simulink library "librnew"  (Simulink 4.00)
undefined symbols (not defined in the file or in its folder): eyediasi, eyesampl, sbiterr, seed

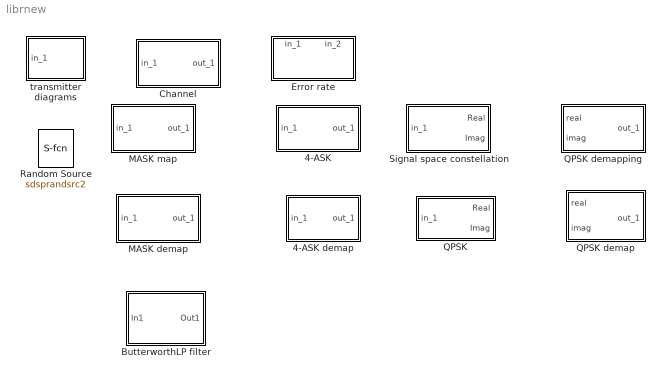
== system librnew ==
  4-ASK : Subsystem  mask(M-ASK mapping){N=4, td=1}
      mask prompts: N "M-ary number (input integers in range [0, M-1]):"; td "Input symbol interval and offset (sec):"
      mask help:
      | Map a digital symbol onto an analog
      | signal in the range [-1, 1] using M-ary
      | amplitude shift keying modulation mapping.
      mask init:
      | Ac=1;Kc=Ac*2/(N-1);
      settings: RTWFcnNameOpts=Auto  RTWFileNameOpts=Auto
      mask Help: This block maps an input digit signal onto a signal in the range [-1, 1]. The coded signal can be modulated using analog\nmodulation blocks. Input digits are in the range [0, M-1], where M is the M-ary number. The input symbol interval can be a two-element vector with the second element being offset. The default value offset is 0. Use the MODMAP function to see the constellation.
      mask Display: disp('MASK\nmapping')
  4-ASK demap : Subsystem  mask(MASK demapping){N=4, td=[1, .9]}
      mask prompts: N "M-ary number (digit integers in ranger [0, M-1]):"; td "Output symbol interval and offset (sec):"
      mask help:
      | Reverse the MASK mapping process
      | Convert [-1 1] analog signal to [0, M-1] symbols.
      mask init:
      | Ac=1;sft=[0:N-1]*Ac*2/(N-1)-Ac;
      settings: RTWFcnNameOpts=Auto  RTWFileNameOpts=Auto
      mask Help: This block demaps a MASK mapped signal back to digit symbols. You can place this block after a amplitude demodulation block. The input of this block is an analog signal in the range [-1, 1]. The demodulation decides the closest integer fitting in [0,M-1] range. When the input symbol interval is a two-elements vector, the second element is offset. The default offset value is 0.
      mask Display: disp('MASK\ndemapping')
  ButterworthLP filter : Subsystem  mask(Lowpass Butterworth filter){n=4}
      mask prompts: n "Cutoff frequency (rad/s)"
      mask init:
      | z = @1 * [];
      | p = @1 * exp(i*(pi*(1:2:n-1)/(2*n) + pi/2));
      | p = [p; conj(p)];
      | p = p(:);
      | if rem(n,2)==1   % n is odd
      |     p = [p; -1];
      | end
      | k = real(prod(-p));
      settings: RTWFcnNameOpts=Auto  RTWFileNameOpts=Auto
      mask Display: plot(0,0,100,100,[90,10,10],[10,10,90],[70,40,9],[10,70,70])
  Channel : Subsystem  mask(AWGN channel, fixed parameter){m=0, variance=0.00010, s=12345}
      mask prompts: m "Mean value:"; variance "Variance (std^2):"; s "Initial Seed:"
      mask help:
      | Additive white Gaussian noise channel
      | with fixed mean and variance.
      mask init:
      | [m,variance,s]=gwnoise(m,variance,s);
      settings: RTWFcnNameOpts=Auto  RTWFileNameOpts=Auto
      mask Help: This block adds white Gaussian noise to the input signal. The mean and the variance can be a scalar or vector with the same length as the input signal.
      mask Display:
      | plot(0,0,100,100);
      | disp('AWGN')
  Error rate : Subsystem  Orientation=down  LoadFcn=sbiterr([],[],[],'LoadBlock')  StartFcn=sbiterr([],[],[],'Start')  StopFcn=sbiterr([],[],[],'Stop')  mask(Symbol/bit error counter){@1=1, @2=10, @3=12, @4=1}
      mask prompts: @1 "Bit per symbol:"; @2 "Number of digits on display:"; @3 "Delay between 1st port and 2nd port:"; @4 "Sample time (sec):"
      mask help: Use the input data from the 1st port as the reference signal to detect the number of errors and error rate of the 2nd signal.
      mask init:
      | K=@1;num_lin=@2;TDelay=@3;Sample=@4;
      settings: CopyFcn=sbiterr([],[],[],'CopyBlock')  DeleteFcn=sbiterr([],[],[],'DeleteBlock')  NameChangeFcn=sbiterr([],[],[],'NameChange')  RTWFcnNameOpts=Auto  RTWFileNameOpts=Auto
      mask Help: The signal from the first port must be a scalar. The second input port can be a vector with a delay to the first port signal. The comparison happens only at the sampling point.
      mask Display: disp('Error\nmeter')
  MASK demap : Subsystem  mask(MASK demap){@1=4, @2=[1, .9]}
      mask prompts: @1 "M-ary number (digit integers in ranger [0, M-1]):"; @2 "Output symbol interval and offset (sec):"
      mask help:
      | Reverse the MASK mapping process
      | Convert [-1 1] analog signal to [0, M-1] symbols.
      mask init:
      | N=@1;Ac=1;sft=[0:N-1]*Ac*2/(N-1)-Ac;td=@2;
      settings: RTWFcnNameOpts=Auto  RTWFileNameOpts=Auto
      mask Help: This block demaps a MASK mapped signal back to digit symbols. You can place this block after a amplitude demodulation block. The input of this block is an analog signal in the range [-1, 1]. The demodulation decides the closest integer fitting in [0,M-1] range. When the input symbol interval is a two-elements vector, the second element is offset. The default offset value is 0.
      mask Display: disp('MASK\ndemap')
  MASK map : Subsystem  mask(MASK map){@1=4, @2=1}
      mask prompts: @1 "M-ary number (input integers in range [0, M-1]):"; @2 "Input symbol interval and offset (sec):"
      mask help:
      | Map a digital symbol onto an analog
      | signal in the range [-1, 1] using M-ary
      | amplitude shift keying modulation mapping.
      mask init:
      | N=@1;Ac=1;Kc=Ac*2/(N-1);td=@2;
      settings: RTWFcnNameOpts=Auto  RTWFileNameOpts=Auto
      mask Help: This block maps an input digit signal onto a signal in the range [-1, 1]. The coded signal can be modulated using analog\nmodulation blocks. Input digits are in the range [0, M-1], where M is the M-ary number. The input symbol interval can be a two-element vector with the second element being offset. The default value offset is 0. Use the MODMAP function to see the constellation.
      mask Display: disp('MASK\nmap')
  QPSK : Subsystem  mask(MPSK){N=[4], A=[sqrt(2)], P=[pi/4], td=1}
      mask prompts: N "Number of symbols in each circle NIC:"; A "Radii in each circle RIC:"; P "Phase shift in each circle PIC (rad):"; td "Symbol interval and offset (sec):"
      mask help: QASK mapping with circle constellation. The constellation is defined in NIC, RIC and PIC.
      mask init:
      | y1=apkconst(N,A,P);y1=[y1;y1];y1=y1(:);y2=imag(y1);y1=real(y1);x=[-sum(N) 1:sum(N)-1;1:sum(N)-1 10*sum(N)]-.5;x=x(:);
      settings: RTWFcnNameOpts=Auto  RTWFileNameOpts=Auto
      mask Help: This block maps a digital signal onto in-phase and quadratic components, which are outputs in the first and second output port respectively. The circle constellation is defined in NIC, RIC, and PIC. The input symbol interval can be a two-element vector with the second element being offset. The default value offset is 0. Use the MODMAP function to see the constellation.
      mask Display: disp('MPSK\nmapping')
  QPSK demap : Subsystem  mask(MPSK demapping){N=[4], A=[sqrt(2)], P=[pi/4], td=1}
      mask prompts: N "Number of symbols on each circle NIC::"; A "Radii for each circle RIC:"; P "Phase shift on each circle PIC (rad):"; td "Symbol interval and offset (sec):"
      mask help:
      | Reverse the QASK map. Input in-phase
      | and quadrature components from the
      | two inputs. Output demapped signal.
      mask init:
      | y1=apkconst(N,A,P);y2=imag(y1);y1=real(y1);
      settings: RTWFcnNameOpts=Auto  RTWFileNameOpts=Auto
      mask Help: This block demaps a QASK mapped signal using circle constellation. You can place this block after a QAM demodulation block. The circle constellation is defined in NIC, RIC, and PIC. The symbol interval can be a two elements vector with the first element being offset. The default offset is zero. Use function MODMAP to view the constellation.
      mask Display: disp('MPSK\ndemapping')
  QPSK demapping : Subsystem  mask(QASK C-demap){@1=[4], @2=[sqrt(2)], @3=[pi/4], @4=1}
      mask prompts: @1 "Number of symbols on each circle NIC::"; @2 "Radii for each circle RIC:"; @3 "Phase shift on each circle PIC (rad):"; @4 "Symbol interval and offset (sec):"
      mask help:
      | Reverse the QASK map. Input in-phase
      | and quadrature components from the
      | two inputs. Output demapped signal.
      mask init:
      | N=@1;A=@2;P=@3;td=@4;y1=apkconst(N,A,P);y2=imag(y1);y1=real(y1);
      settings: RTWFcnNameOpts=Auto  RTWFileNameOpts=Auto
      mask Help: This block demaps a QASK mapped signal using circle constellation. You can place this block after a QAM demodulation block. The circle constellation is defined in NIC, RIC, and PIC. The symbol interval can be a two elements vector with the first element being offset. The default offset is zero. Use function MODMAP to view the constellation.
      mask Display: disp('QASK\nC-demap')
  Random Source : S-Function  FunctionName=sdsprandsrc2  Parameters=SrcType,Min,Max,Mean,Var,SFcnSeed,Inherit,SampMode,SampTime,SampFrame,OutComplex,RepMode,Seed  PortCounts=[]  SFunctionModules=''  mask(Random Source){SrcType=Gaussian, Min=0, Max=1, Mean=0, Var=1, RepMode=Specify seed, Seed=seed, Inherit=on, SampMode=Discrete, SampTime=1, SampFrame=1, OutComplex=Real}
      mask prompts: SrcType "Source type:"; Min "Minimum:"; Max "Maximum:"; Var "Variance:"; RepMode "Repeatability:"; Seed "Initial seed:"; Inherit "Inherit output port attributes"; SampMode "Sample mode:"; SampTime "Sample time:"; SampFrame "Samples per frame:"; OutComplex "Output complexity:"
      mask help: Output a random signal with uniform or Gaussian (normal) distribution. Set output repeatability to Nonrepeatable (block randomly selects initial seed every time simulation starts), Repeatable (block randomly selects initial seed once and uses it every time simulation starts), or Specify seed (block uses specified initial seed every time simulation starts, producing repeatable output).
      mask init:
      | [x,y]=dspblkrandsrc2('icon');SFcnSeed=eval(dspblkrandsrc2('seed'),'Seed');
      mask Help: web(dspbhelp);
      mask StyleString: popup(Uniform|Gaussian),edit,edit,edit,edit,popup(Specify seed|Repeatable|Not repeatable),edit,checkbox,popup(Discrete|Continuous),edit,edit,popup(Real|Complex)
      mask CallbackString: dspblkrandsrc2;|||||dspblkrandsrc2;||dspblkrandsrc2;|dspblkrandsrc2;|||
      mask Display: plot(x,y);
  Signal space constellation : Subsystem  mask(QASK C-map){@1=[4], @2=[sqrt(2)], @3=[pi/4], @4=1}
      mask prompts: @1 "Number of symbols in each circle NIC:"; @2 "Radii in each circle RIC:"; @3 "Phase shift in each circle PIC (rad):"; @4 "Symbol interval and offset (sec):"
      mask help: QASK mapping with circle constellation. The constellation is defined in NIC, RIC and PIC.
      mask init:
      | N=@1;A=@2;P=@3;td=@4;y1=apkconst(N,A,P);y1=[y1;y1];y1=y1(:);y2=imag(y1);y1=real(y1);x=[-sum(N) 1:sum(N)-1;1:sum(N)-1 10*sum(N)]-.5;x=x(:);
      settings: RTWFcnNameOpts=Auto  RTWFileNameOpts=Auto
      mask Help: This block maps a digital signal onto in-phase and quadratic components, which are outputs in the first and second output port respectively. The circle constellation is defined in NIC, RIC, and PIC. The input symbol interval can be a two-element vector with the second element being offset. The default value offset is 0. Use the MODMAP function to see the constellation.
      mask Display: disp('QASK\nC-map')
  transmitter diagrams : Subsystem  mask(Diagrams){starttime=6, anzahl=40, offset=0}
      mask prompts: starttime "Plot start time:"; anzahl "samples per time slot"; offset "decision offset"
      mask help: Eye pattern, signal-space trajectory and scatter plot
      mask init:
      | [x, y] = srcsicon(10);
      settings: RTWFcnNameOpts=Auto  RTWFileNameOpts=Auto
      mask Display: plot(0,0,100,100,x,y)

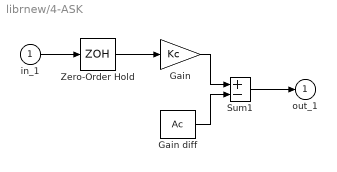
== system librnew/4-ASK ==
  in_1 : Inport  Port=1  LatchInput=off
  Gain : Gain  Gain=Kc  Multiplication=Element-wise(K.*u)  SaturateOnIntegerOverflow=on
  Gain diff : Constant  Value=Ac
  Sum1 : Sum  Inputs=+-  SaturateOnIntegerOverflow=on
  Zero-Order Hold : ZeroOrderHold  SampleTime=td
  out_1 : Outport  Port=1
  wires:
  Gain/1 -> Sum1/1
  Gain diff/1 -> Sum1/2
  Sum1/1 -> out_1/1
  in_1/1 -> Zero-Order Hold/1
  Zero-Order Hold/1 -> Gain/1

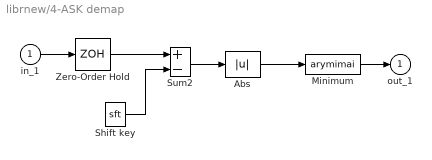
== system librnew/4-ASK demap ==
  in_1 : Inport  Port=1  LatchInput=off
  Abs : Abs  SaturateOnIntegerOverflow=on
  Minimum : S-Function  FunctionName=arymimai  Parameters='min'  PortCounts=[]  SFunctionModules=''
  Shift key : Constant  Value=sft
  Sum2 : Sum  Inputs=+-  SaturateOnIntegerOverflow=on
  Zero-Order Hold : ZeroOrderHold  SampleTime=td
  out_1 : Outport  Port=1
  wires:
  in_1/1 -> Zero-Order Hold/1
  Abs/1 -> Minimum/1
  Zero-Order Hold/1 -> Sum2/1
  Minimum/1 -> out_1/1
  Shift key/1 -> Sum2/2
  Sum2/1 -> Abs/1

== system librnew/ButterworthLP filter ==
  In1 : Inport  Port=1  LatchInput=off
  Zero-Pole : ZeroPole  Zeros=z  Poles=p  Gain=k  AbsoluteTolerance=auto
  Out1 : Outport  Port=1
  wires:
  Zero-Pole/1 -> Out1/1
  In1/1 -> Zero-Pole/1

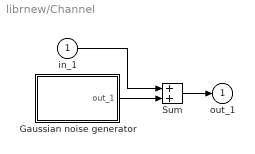
== system librnew/Channel ==
  in_1 : Inport  Port=1  LatchInput=off
  Gaussian noise generator : Subsystem  mask(Gaussian noise generator){m=m, variance=variance, s=s}
      mask prompts: m "Mean value:"; variance "Variance (vector or matrix):"; s "Initial seed:"
      mask help:
      | Generate Gaussian distributed noise with
      | given mean and variance value.
      mask init:
      | [m,variance,s]=gwnoise(m,variance,s);[x,y]=srcsicon(3);
      settings: RTWFcnNameOpts=Auto  RTWFileNameOpts=Auto
      mask Help: When the mean value and seed are vectors, the output of this block is a vector. The length of the vector is the same as the length of the mean value vector or the length of the seed. When the variance entry is a vector, the variance is a diagonal matrix.
      mask Display: plot(0,0,100,100,x,y);disp('Gaussian')
  Sum : Sum  Inputs=++  SaturateOnIntegerOverflow=on
  out_1 : Outport  Port=1
  wires:
  Sum/1 -> out_1/1
  in_1/1 -> Sum/1
  Gaussian noise generator/1(out_1) -> Sum/2

== system librnew/Error rate ==
  in_1 : Inport  Port=1  LatchInput=off
  in_2 : Inport  Port=2  LatchInput=off
  Mux : Mux  Inputs=2
      settings: DisplayOption=none
  S-function : S-Function  FunctionName=sbiterr  Parameters=num_lin, K, TDelay, Sample  PortCounts=[]  SFunctionModules=''
  wires:
  Mux/1 -> S-function/1
  in_1/1 -> Mux/1
  in_2/1 -> Mux/2

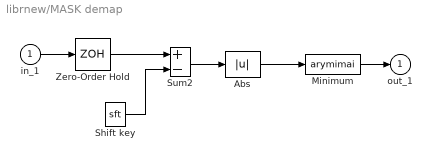
== system librnew/MASK demap ==
  in_1 : Inport  Port=1  LatchInput=off
  Abs : Abs  SaturateOnIntegerOverflow=on
  Minimum : S-Function  FunctionName=arymimai  Parameters='min'  PortCounts=[]  SFunctionModules=''
  Shift key : Constant  Value=sft
  Sum2 : Sum  Inputs=+-  SaturateOnIntegerOverflow=on
  Zero-Order Hold : ZeroOrderHold  SampleTime=td
  out_1 : Outport  Port=1
  wires:
  in_1/1 -> Zero-Order Hold/1
  Abs/1 -> Minimum/1
  Zero-Order Hold/1 -> Sum2/1
  Minimum/1 -> out_1/1
  Shift key/1 -> Sum2/2
  Sum2/1 -> Abs/1

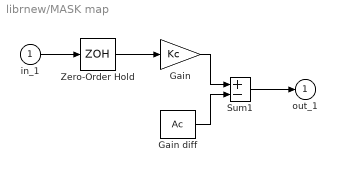
== system librnew/MASK map ==
  in_1 : Inport  Port=1  LatchInput=off
  Gain : Gain  Gain=Kc  Multiplication=Element-wise(K.*u)  SaturateOnIntegerOverflow=on
  Gain diff : Constant  Value=Ac
  Sum1 : Sum  Inputs=+-  SaturateOnIntegerOverflow=on
  Zero-Order Hold : ZeroOrderHold  SampleTime=td
  out_1 : Outport  Port=1
  wires:
  Gain/1 -> Sum1/1
  Gain diff/1 -> Sum1/2
  Sum1/1 -> out_1/1
  in_1/1 -> Zero-Order Hold/1
  Zero-Order Hold/1 -> Gain/1

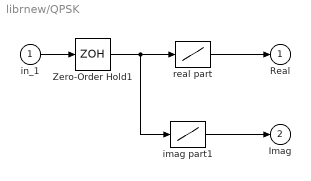
== system librnew/QPSK ==
  in_1 : Inport  Port=1  LatchInput=off
  Zero-Order Hold1 : ZeroOrderHold  SampleTime=td
  imag part1 : Lookup  InputValues=x  OutputValues=y2
  real part : Lookup  InputValues=x  OutputValues=y1
  Real : Outport  Port=1
  Imag : Outport  Port=2
  wires:
  in_1/1 -> Zero-Order Hold1/1
  Zero-Order Hold1/1 -> real part/1, imag part1/1
  real part/1 -> Real/1
  imag part1/1 -> Imag/1

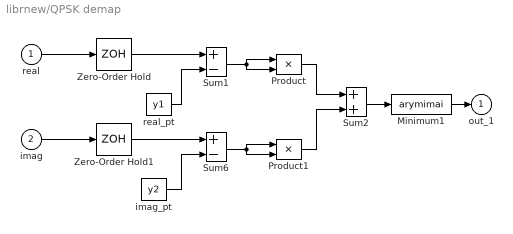
== system librnew/QPSK demap ==
  real : Inport  Port=1  LatchInput=off
  imag : Inport  Port=2  LatchInput=off
  Minimum1 : S-Function  FunctionName=arymimai  Parameters='min'  PortCounts=[]  SFunctionModules=''
  Product : Product  Inputs=2  Multiplication=Element-wise(.*)  SaturateOnIntegerOverflow=on
  Product1 : Product  Inputs=2  Multiplication=Element-wise(.*)  SaturateOnIntegerOverflow=on
  Sum1 : Sum  Inputs=+-  SaturateOnIntegerOverflow=on
  Sum2 : Sum  Inputs=++  SaturateOnIntegerOverflow=on
  Sum6 : Sum  Inputs=+-  SaturateOnIntegerOverflow=on
  Zero-Order Hold : ZeroOrderHold  SampleTime=td
  Zero-Order Hold1 : ZeroOrderHold  SampleTime=td
  imag_pt : Constant  Value=y2
  real_pt : Constant  Value=y1
  out_1 : Outport  Port=1
  wires:
  Minimum1/1 -> out_1/1
  Sum2/1 -> Minimum1/1
  Product1/1 -> Sum2/2
  Product/1 -> Sum2/1
  Sum6/1 -> Product1/2, Product1/1
  Sum1/1 -> Product/2, Product/1
  imag_pt/1 -> Sum6/2
  Zero-Order Hold1/1 -> Sum6/1
  Zero-Order Hold/1 -> Sum1/1
  real_pt/1 -> Sum1/2
  imag/1 -> Zero-Order Hold1/1
  real/1 -> Zero-Order Hold/1

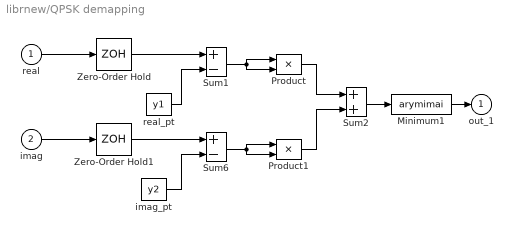
== system librnew/QPSK demapping ==
  real : Inport  Port=1  LatchInput=off
  imag : Inport  Port=2  LatchInput=off
  Minimum1 : S-Function  FunctionName=arymimai  Parameters='min'  PortCounts=[]  SFunctionModules=''
  Product : Product  Inputs=2  Multiplication=Element-wise(.*)  SaturateOnIntegerOverflow=on
  Product1 : Product  Inputs=2  Multiplication=Element-wise(.*)  SaturateOnIntegerOverflow=on
  Sum1 : Sum  Inputs=+-  SaturateOnIntegerOverflow=on
  Sum2 : Sum  Inputs=++  SaturateOnIntegerOverflow=on
  Sum6 : Sum  Inputs=+-  SaturateOnIntegerOverflow=on
  Zero-Order Hold : ZeroOrderHold  SampleTime=td
  Zero-Order Hold1 : ZeroOrderHold  SampleTime=td
  imag_pt : Constant  Value=y2
  real_pt : Constant  Value=y1
  out_1 : Outport  Port=1
  wires:
  Minimum1/1 -> out_1/1
  Sum2/1 -> Minimum1/1
  Product1/1 -> Sum2/2
  Product/1 -> Sum2/1
  Sum6/1 -> Product1/1, Product1/2
  Sum1/1 -> Product/1, Product/2
  imag_pt/1 -> Sum6/2
  Zero-Order Hold1/1 -> Sum6/1
  Zero-Order Hold/1 -> Sum1/1
  real_pt/1 -> Sum1/2
  imag/1 -> Zero-Order Hold1/1
  real/1 -> Zero-Order Hold/1

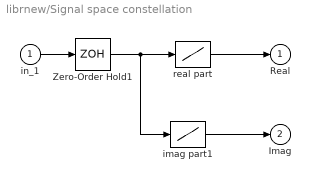
== system librnew/Signal space constellation ==
  in_1 : Inport  Port=1  LatchInput=off
  Zero-Order Hold1 : ZeroOrderHold  SampleTime=td
  imag part1 : Lookup  InputValues=x  OutputValues=y2
  real part : Lookup  InputValues=x  OutputValues=y1
  Real : Outport  Port=1
  Imag : Outport  Port=2
  wires:
  in_1/1 -> Zero-Order Hold1/1
  Zero-Order Hold1/1 -> imag part1/1, real part/1
  real part/1 -> Real/1
  imag part1/1 -> Imag/1

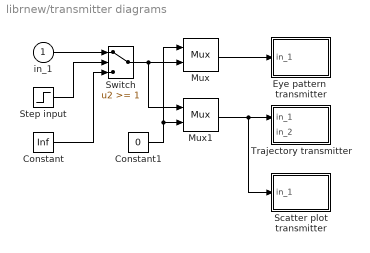
== system librnew/transmitter diagrams ==
  in_1 : Inport  Port=1  LatchInput=off
  Constant : Constant  Value=Inf
  Constant1 : Constant  Value=0
  Eye pattern  transmitter : Subsystem  LoadFcn=eyesampl([],[],[],'LoadBlock')  StartFcn=eyesampl([],[],[],'Start')  StopFcn=eyesampl([],[],[],'Stop')  mask(Eye-diagram/scatter plot){@1=[2 0 1+offset], @2=[-1.5 1.5], @3=0, @4='w-/r-', @5=0, @6=2/anzahl}
      mask prompts: @1 "[Symbol interval, plot offset, decision point offset]:"; @2 "Lower and upper bound of in-coming signal (1x2 vector):"; @3 "Number of saved traces:"; @4 "Line-type for eye-pattern diagram (0 for no plot):"; @5 "Line-type for scatter plot (0 for no plot):"; @6 "Plot update sample time:"
      mask help: Produce eye-pattern diagram and/or scatter plot.
      mask init:
      | time_range=@1;boundary=@2;kept_length=@3;eye_line=@4;scatter_line=@5;two_d_line=@6;[x,y]=srcsicon(10);
      settings: CopyFcn=eyesampl([],[],[],'CopyBlock')  DeleteFcn=eyesampl([],[],[],'DeleteBlock')  NameChangeFcn=eyesampl([],[],[],'NameChange')  RTWFcnNameOpts=Auto  RTWFileNameOpts=Auto
      mask Help: This plot opens one, or two plots by assigning the line type parameters. The scatter plot point is selected by the decision point in the first parameter entry. A decision line is drawn in the eye-pattern diagram. The plot is updated at the plot update sample time point.
      mask Display: plot(0,0,100,100,x,y);
  Mux : Mux  Inputs=2
      settings: DisplayOption=none
  Mux1 : Mux  Inputs=2
      settings: DisplayOption=none
  Scatter plot transmitter : Subsystem  LoadFcn=eyesampl([],[],[],'LoadBlock')  StartFcn=eyesampl([],[],[],'Start')  StopFcn=eyesampl([],[],[],'Stop')  mask(Eye-diagram/scatter plot){@1=[1 .5 .999], @2=[-1.5 1.5], @3=0, @4=0, @5='b.', @6=[.5 offset]}
      mask prompts: @1 "[Symbol interval, plot offset, decision point offset]:"; @2 "Lower and upper bound of in-coming signal (1x2 vector):"; @3 "Number of saved traces:"; @4 "Line-type for eye-pattern diagram (0 for no plot):"; @5 "Line-type for scatter plot (0 for no plot):"; @6 "Plot update sample time:"
      mask help: Produce eye-pattern diagram and/or scatter plot.
      mask init:
      | time_range=@1;boundary=@2;kept_length=@3;eye_line=@4;scatter_line=@5;two_d_line=@6;[x,y]=srcsicon(10);
      settings: CopyFcn=eyesampl([],[],[],'CopyBlock')  DeleteFcn=eyesampl([],[],[],'DeleteBlock')  NameChangeFcn=eyesampl([],[],[],'NameChange')  RTWFcnNameOpts=Auto  RTWFileNameOpts=Auto
      mask Help: This plot opens one, or two plots by assigning the line type parameters. The scatter plot point is selected by the decision point in the first parameter entry. A decision line is drawn in the eye-pattern diagram. The plot is updated at the plot update sample time point.
      mask Display: plot(0,0,100,100,x,y);
  Step input : Step  Time=starttime  Before=0  After=1  SampleTime=1
  Switch : Switch  Threshold=1
  Trajectory transmitter : Subsystem  LoadFcn=eyediasi([],[],[],'LoadBlock')  StartFcn=eyediasi([],[],[],'Start')  StopFcn=eyediasi([],[],[],'Stop')  mask(Eye-diagram/scatter plot){@1=[2 0 1], @2=[-1.5 1.5], @3=0, @4=0, @5=0, @6='g-'}
      mask prompts: @1 "Eye-pattern plot time frame:"; @2 "Lower and upper bound of in-coming signal (1x2 vector):"; @3 "Number of saved traces:"; @4 "Line-type for eye-pattern diagram (0 for no plot):"; @5 "Line-type for scatter plot (0 for no plot):"; @6 "Line-type for x-y plot (0 for no plot):"
      mask help:
      | Produce eye-pattern diagram/scatter
      | plot/x-y plot with the rising edge of the second input as the decision line.
      mask init:
      | time_range=@1;boundary=@2;kept_length=@3;eye_line=@4;scatter_line=@5;two_d_line=@6;[x,y]=srcsicon(10);[v,w]=trigicon(0,25,get_param(gcb,'orientation'),2);
      settings: CopyFcn=eyediasi([],[],[],'CopyBlock')  DeleteFcn=eyediasi([],[],[],'DeleteBlock')  NameChangeFcn=eyediasi([],[],[],'NameChange')  RTWFcnNameOpts=Auto  RTWFileNameOpts=Auto
      mask Help: This plot opens one, two, or three plots by assigning the line type parameters. The scatter plot point is selected by the rising edge of a trigger signal. A decision line is drawn at the rising edge of the trigger signal.
      mask Display: plot(0,0,100,100,x,y,v,w);
  wires:
  Mux/1 -> Eye pattern  transmitter/1(in_1)
  in_1/1 -> Switch/1
  Step input/1 -> Switch/2
  Constant/1 -> Switch/3
  Mux1/1 -> Scatter plot transmitter/1(in_1), Trajectory transmitter/1(in_1)
  Constant1/1 -> Mux1/2, Mux/1
  Switch/1 -> Mux1/1, Mux/2

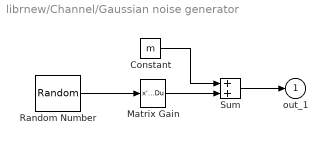
== system librnew/Channel/Gaussian noise generator ==
  Constant : Constant  Value=m
  Matrix Gain : StateSpace  A=[]  B=[]  C=[]  D=K  X0=0  AbsoluteTolerance=auto  Realization=auto  mask(Matrix Gain){@1=variance}
      mask prompts: @1 "Gain matrix:"
      mask help: Matrix Gain.
      mask init:
      | K = @1;
      mask Help: Multiplies input vector by entered matrix to produce output vector (y=Au).
      mask Display: disp('K')
  Random Number : RandomNumber  Mean=0  Variance=1  Seed=s  SampleTime=0
  Sum : Sum  Inputs=++  SaturateOnIntegerOverflow=on
  out_1 : Outport  Port=1
  wires:
  Constant/1 -> Sum/1
  Sum/1 -> out_1/1
  Matrix Gain/1 -> Sum/2
  Random Number/1 -> Matrix Gain/1

== system librnew/transmitter diagrams/Eye pattern  transmitter ==
  in_1 : Inport  Port=1  LatchInput=off
  Plot1 : S-Function  FunctionName=eyesampl  Parameters=time_range, boundary, kept_length, eye_line, scatter_line, two_d_line  PortCounts=[]  SFunctionModules=''
  wires:
  in_1/1 -> Plot1/1

== system librnew/transmitter diagrams/Scatter plot transmitter ==
  in_1 : Inport  Port=1  LatchInput=off
  Plot1 : S-Function  FunctionName=eyesampl  Parameters=time_range, boundary, kept_length, eye_line, scatter_line, two_d_line  PortCounts=[]  SFunctionModules=''
  wires:
  in_1/1 -> Plot1/1

== system librnew/transmitter diagrams/Trajectory transmitter ==
  in_1 : Inport  Port=1  LatchInput=off
  in_2 : Inport  Port=2  LatchInput=off
  Mux : Mux  Inputs=2
      settings: DisplayOption=none
  Plot1 : S-Function  FunctionName=eyediasi  Parameters=time_range, boundary, kept_length, eye_line, scatter_line, two_d_line  PortCounts=[]  SFunctionModules=''
  wires:
  Mux/1 -> Plot1/1
  in_2/1 -> Mux/2
  in_1/1 -> Mux/1
